simulink model "Height_Diff_SS_D_1"  (R2013a)
settings: Solver=ode45  StartTime=0.0  StopTime=30  RelTol=1e-3
values from neighbouring files (symbols this model uses):
  A_Height_d = [1  0.02  0.00306066709295; 0  1  0.292172619905; 0  0  0.751477293075]    [Height_Controller_SS_D_Data.mat]
  B_Height_d = [0.000298297262238 0.0437238156136 0.248522706925]    [Height_Controller_SS_D_Data.mat]
  C_Height_d = [1 0 0]    [Height_Controller_SS_D_Data.mat]
  F_yIntercept = -10.4432883127    [Model_Parameters.mat]
  Feed_Forward_Height_d = 2    [Height_Controller_SS_D_Data.mat]
  g = 9.81    [Model_Parameters.mat]
  G_Height_d = [1.74010652855 42.1423339094 13.9880450099]    [Height_Controller_SS_D_Data.mat]
  K_Height_d = [2.48783179706 0.673217306935 0.6059224462]    [Height_Controller_SS_D_Data.mat]
  K_Height_i = -2.04253032079    [Height_Controller_SS_D_Data.mat]
  Kf = 9.48907430341    [Model_Parameters.mat]
  Mass = 2.26    [Model_Parameters.mat]
  Motor_TimeConstant = 0.07    [Model_Parameters.mat]
  Ts = 20e-3    (= 0.02)    [All_Controller_Sample_Time.m]
undefined symbols (not defined in the file or in its folder): DiscIntNeverNeededParam
libraries: simulink x2
settings Model: Creator=Ross  LastModifiedBy=Ross

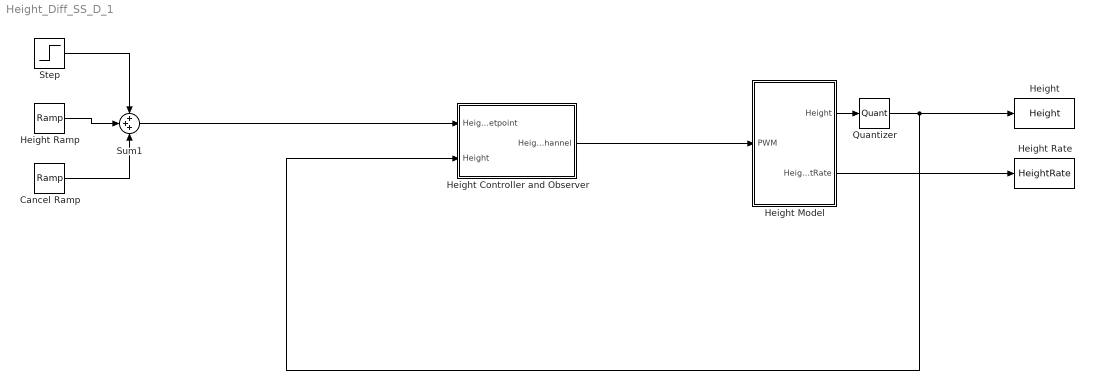
== system Height_Diff_SS_D_1 ==
  Cancel Ramp : simulink/Sources/Ramp  slope=-1  start=2  X0=0
  Height : ToWorkspace  VariableName=Height  SampleTime=-1  SaveFormat=Timeseries
  Height Ramp : simulink/Sources/Ramp  slope=1  start=1  X0=0
  Height Controller and Observer : Subsystem
  Height Model : Subsystem
  Height Rate : ToWorkspace  VariableName=HeightRate  SampleTime=-1  SaveFormat=Timeseries
  Quantizer : Quantizer  QuantizationInterval=0.01
  Step : Step  Time=10  SampleTime=0
  Sum1 : Sum  Inputs=+++
  wires:
  Sum1/1 -> Height Controller and Observer/1(Height Setpoint)
  Step/1 -> Sum1/1
  Height Ramp/1 -> Sum1/2
  Cancel Ramp/1 -> Sum1/3
  Height Model/2(HeightRate) -> Height Rate/1
  Height Model/1(Height) -> Quantizer/1
  Height Controller and Observer/1(Height Channel) -> Height Model/1(PWM)
  Quantizer/1 -> Height/1, Height Controller and Observer/2(Height)

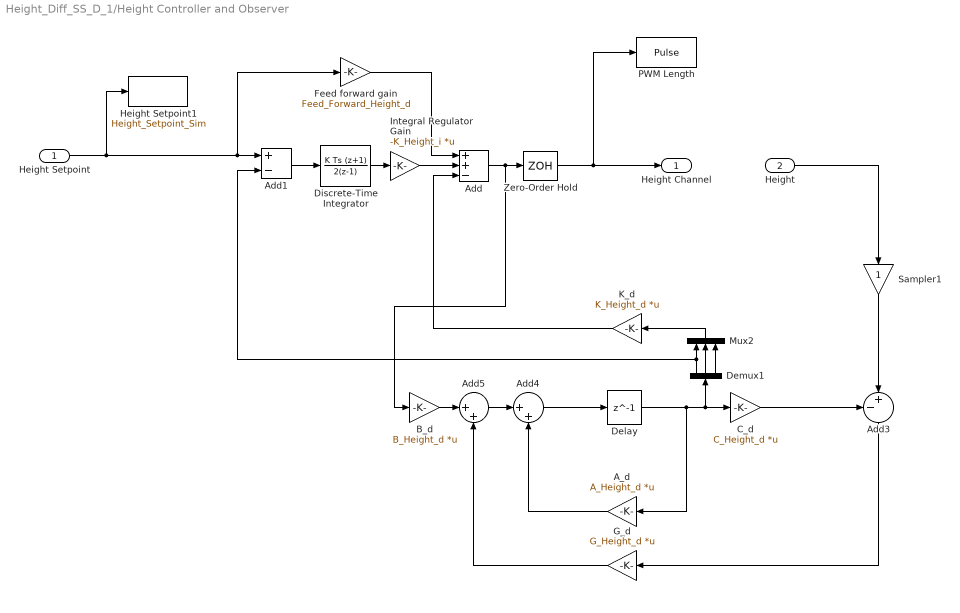
== system Height_Diff_SS_D_1/Height Controller and Observer ==
  Height Setpoint : Inport
  Height : Inport  Port=2
  A_d : Gain  Gain=A_Height_d  Multiplication=Matrix(K*u)  SampleTime=Ts
  Add : Sum  Inputs=++-
  Add1 : Sum  Inputs=+-
  Add3 : Sum  Inputs=-+|
  Add4 : Sum  Inputs=|++
  Add5 : Sum  Inputs=|++
  "B_d " : Gain  Gain=B_Height_d  Multiplication=Matrix(K*u)  SampleTime=Ts
  "C_d " : Gain  Gain=C_Height_d  Multiplication=Matrix(K*u)  SampleTime=Ts
  Delay : Delay  DelayLength=1  InitialCondition=0  SampleTime=Ts
  Demux1 : Demux  Outputs=3
  Discrete-Time Integrator : DiscreteIntegrator  IntegratorMethod=Integration: Trapezoidal  gainval=1  SampleTime=Ts  ICPrevOutput=DiscIntNeverNeededParam  ICPrevScaledInput=DiscIntNeverNeededParam
  Feed forward gain : Gain  Gain=Feed_Forward_Height_d  SampleTime=Ts
  G_d : Gain  Gain=G_Height_d  Multiplication=Matrix(K*u)  SampleTime=Ts
  Height Setpoint1 : ToWorkspace  VariableName=Height_Setpoint_Sim  SampleTime=-1  SaveFormat=Timeseries
  Integral Regulator Gain : Gain  Gain=-K_Height_i  Multiplication=Matrix(K*u)  SampleTime=Ts
  K_d : Gain  Gain=K_Height_d  Multiplication=Matrix(K*u)  SampleTime=Ts
  Mux2 : Mux  Inputs=3
  PWM Length : ToWorkspace  VariableName=Pulse  SampleTime=-1  SaveFormat=Timeseries
  Sampler1 : Gain  SampleTime=Ts
  Zero-Order Hold : ZeroOrderHold  SampleTime=Ts
  Height Channel : Outport
  wires:
  Add/1 -> "B_d "/1, Zero-Order Hold/1
  "B_d "/1 -> Add5/1
  K_d/1 -> Add/3
  Demux1/2 -> Mux2/2
  Sampler1/1 -> Add3/2
  Add4/1 -> Delay/1
  Add3/1 -> G_d/1
  Demux1/3 -> Mux2/3
  Demux1/1 -> Add1/2, Mux2/1
  G_d/1 -> Add5/2
  Delay/1 -> "C_d "/1, Demux1/1, A_d/1
  Mux2/1 -> K_d/1
  "C_d "/1 -> Add3/1
  A_d/1 -> Add4/2
  Add5/1 -> Add4/1
  Height/1 -> Sampler1/1
  Height Setpoint/1 -> Height Setpoint1/1, Feed forward gain/1, Add1/1
  Zero-Order Hold/1 -> Height Channel/1, PWM Length/1
  Feed forward gain/1 -> Add/1
  Discrete-Time Integrator/1 -> Integral Regulator Gain/1
  Add1/1 -> Discrete-Time Integrator/1
  Integral Regulator Gain/1 -> Add/2

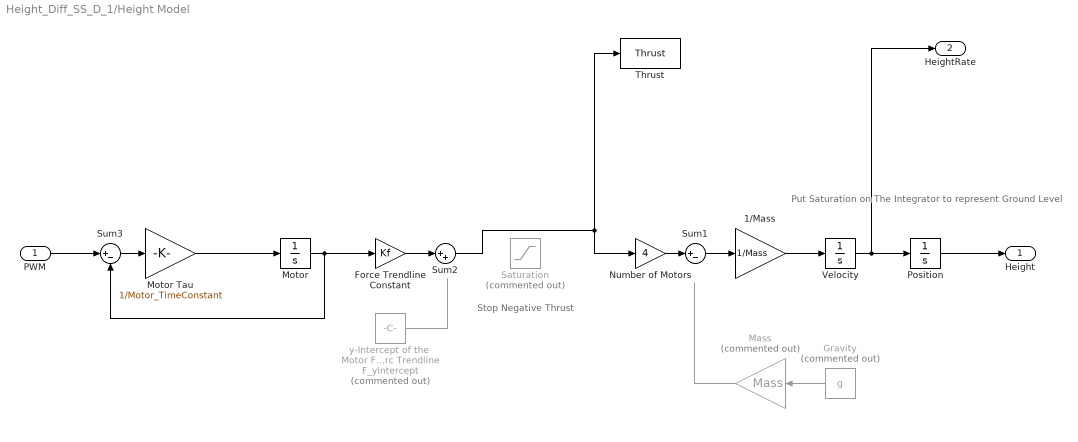
== system Height_Diff_SS_D_1/Height Model ==
  note: Stop Negative
      | Thrust
  note: Put Saturation on
      | The Integrator to represent
      | Ground Level
  PWM : Inport
  1/Mass : Gain  Gain=1/Mass
  Force Trendline Constant : Gain  Gain=Kf
  Gravity : Constant  Commented=on  Value=g
  Mass : Gain  Commented=on  Gain=Mass
  Motor : Integrator
  Motor Tau : Gain  Gain=1/Motor_TimeConstant
  Number of Motors : Gain  Gain=4
  Position : Integrator  LowerSaturationLimit=0
  Saturation : Saturate  Commented=on  UpperLimit=inf  LowerLimit=0
  Sum1 : Sum  Inputs=|+-
  Sum2 : Sum  Inputs=|++
  Sum3 : Sum  Inputs=|+-
  Thrust : ToWorkspace  VariableName=Thrust  SampleTime=-1  SaveFormat=Timeseries
  Velocity : Integrator
  y-Intercept of the  Motor Forc Trendline : Constant  Commented=on  Value=F_yIntercept
  Height : Outport
  HeightRate : Outport  Port=2
  wires:
  Motor Tau/1 -> Motor/1
  Number of Motors/1 -> Sum1/1
  Position/1 -> Height/1
  PWM/1 -> Sum3/1
  Velocity/1 -> HeightRate/1, Position/1
  Sum3/1 -> Motor Tau/1
  1/Mass/1 -> Velocity/1
  Gravity/1 -> Mass/1
  Mass/1 -> ?
  Sum1/1 -> 1/Mass/1
  y-Intercept of the  Motor Forc Trendline/1 -> ?
  Force Trendline Constant/1 -> Sum2/1
  Sum2/1 -> Number of Motors/1, Thrust/1
  Motor/1 -> Sum3/2, Force Trendline Constant/1
